simulink model "simu"  (R2014a)
settings: Solver=ode23t  StartTime=0.0  StopTime=2  FixedStep=0.00001  MaxStep=0.0001  RelTol=1e-3
undefined symbols (not defined in the file or in its folder): param
settings Model: Creator=Etienne  LastModifiedBy=Etienne

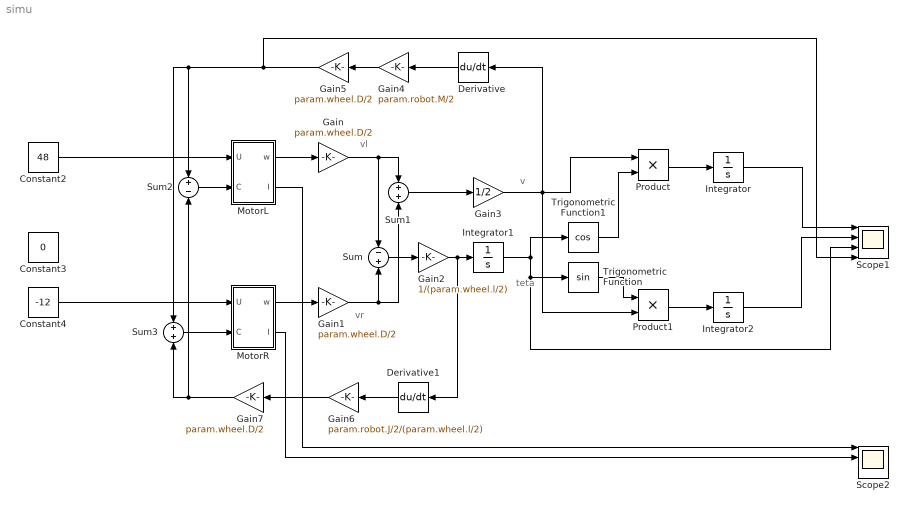
== system simu ==
  note: v
  note: teta
  note: vr
  note: vl
  Constant2 : Constant  Value=48
  Constant3 : Constant  Value=0
  Constant4 : Constant  Value=-12
  Derivative : Derivative
  Derivative1 : Derivative
  Gain{,1,5,7} (4 alike) : Gain  Gain=param.wheel.D/2
  Gain2 : Gain  Gain=1/(param.wheel.l/2)
  Gain3 : Gain  Gain=1/2
  Gain4 : Gain  Gain=param.robot.M/2
  Gain6 : Gain  Gain=param.robot.J/2/(param.wheel.l/2)
  Integrator : Integrator
  Integrator1 : Integrator
  Integrator2 : Integrator
  MotorL : Subsystem
  MotorR : Subsystem
  Product : Product
  Product1 : Product
  Scope1 : Scope  NumInputPorts=4
      settings: TimeRange=2  YMin=-0.06~-0.1~-15~-0.2  YMax=0.06~0.01999999999999999~0~1  MaxDataPoints=5000000
  Scope2 : Scope  NumInputPorts=4
      settings: TimeRange=2  YMin=0~-6~-1~-1  YMax=6~0~1~1  SaveName=ScopeData2  MaxDataPoints=5000000
  Sum : Sum  Inputs=-|+
  Sum1 : Sum  Inputs=+|+
  Sum2 : Sum  Inputs=+|-
  Sum3 : Sum  Inputs=+|+
  Trigonometric Function : Trigonometry
  Trigonometric Function1 : Trigonometry  Operator=cos
  wires:
  Gain/1 -> Sum/1, Sum1/1
  Integrator/1 -> Scope1/1
  MotorR/1(w) -> Gain1/1
  Gain1/1 -> Sum/2, Sum1/2
  Sum/1 -> Gain2/1
  Gain2/1 -> Derivative1/1, Integrator1/1
  Sum1/1 -> Gain3/1
  Gain3/1 -> Derivative/1, Product1/2, Product/1
  Integrator1/1 -> Trigonometric Function1/1, Scope1/3, Trigonometric Function/1
  Trigonometric Function1/1 -> Product/2
  Trigonometric Function/1 -> Product1/1
  Product/1 -> Integrator/1
  Product1/1 -> Integrator2/1
  Integrator2/1 -> Scope1/2
  Constant4/1 -> MotorR/1(U)
  Derivative/1 -> Gain4/1
  Gain4/1 -> Gain5/1
  Gain5/1 -> Sum3/1, Sum2/1, Scope1/4
  MotorR/2(I) -> Scope2/2
  Sum3/1 -> MotorR/2(C)
  Gain6/1 -> Gain7/1
  Gain7/1 -> Sum2/2, Sum3/2
  Derivative1/1 -> Gain6/1
  Constant2/1 -> MotorL/1(U)
  Sum2/1 -> MotorL/2(C)
  MotorL/1(w) -> Gain/1
  MotorL/2(I) -> Scope2/1

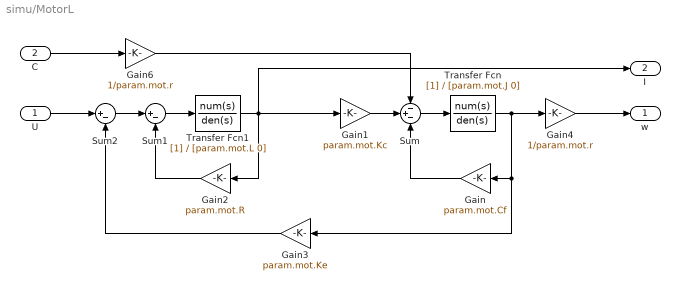
== system simu/MotorL ==
  U : Inport
  C : Inport  Port=2
  Gain : Gain  Gain=param.mot.Cf
  Gain1 : Gain  Gain=param.mot.Kc
  Gain2 : Gain  Gain=param.mot.R
  Gain3 : Gain  Gain=param.mot.Ke
  Gain4 : Gain  Gain=1/param.mot.r
  Gain6 : Gain  Gain=1/param.mot.r
  Sum : Sum  Inputs=-+-
  Sum1 : Sum  Inputs=|+-
  Sum2 : Sum  Inputs=|+-
  Transfer Fcn : TransferFcn  Denominator=[param.mot.J 0]
  Transfer Fcn1 : TransferFcn  Denominator=[param.mot.L 0]
  w : Outport
  I : Outport  Port=2
  wires:
  Gain1/1 -> Sum/2
  Transfer Fcn/1 -> Gain4/1, Gain3/1, Gain/1
  Gain3/1 -> Sum2/2
  Gain/1 -> Sum/3
  Sum2/1 -> Sum1/1
  Gain2/1 -> Sum1/2
  Sum1/1 -> Transfer Fcn1/1
  U/1 -> Sum2/1
  C/1 -> Gain6/1
  Gain6/1 -> Sum/1
  Gain4/1 -> w/1
  Sum/1 -> Transfer Fcn/1
  Transfer Fcn1/1 -> Gain1/1, I/1, Gain2/1

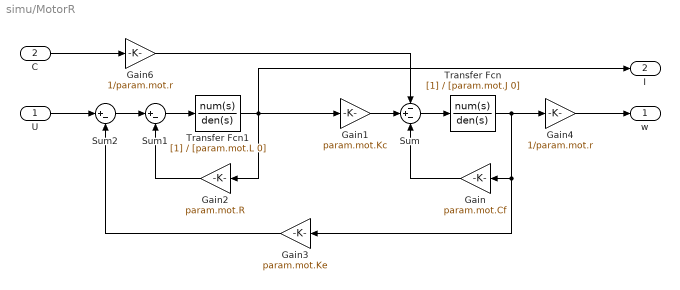
== system simu/MotorR ==
  U : Inport
  C : Inport  Port=2
  Gain : Gain  Gain=param.mot.Cf
  Gain1 : Gain  Gain=param.mot.Kc
  Gain2 : Gain  Gain=param.mot.R
  Gain3 : Gain  Gain=param.mot.Ke
  Gain4 : Gain  Gain=1/param.mot.r
  Gain6 : Gain  Gain=1/param.mot.r
  Sum : Sum  Inputs=-+-
  Sum1 : Sum  Inputs=|+-
  Sum2 : Sum  Inputs=|+-
  Transfer Fcn : TransferFcn  Denominator=[param.mot.J 0]
  Transfer Fcn1 : TransferFcn  Denominator=[param.mot.L 0]
  w : Outport
  I : Outport  Port=2
  wires:
  Gain1/1 -> Sum/2
  Transfer Fcn/1 -> Gain4/1, Gain3/1, Gain/1
  Gain3/1 -> Sum2/2
  Gain/1 -> Sum/3
  Sum2/1 -> Sum1/1
  Gain2/1 -> Sum1/2
  Sum1/1 -> Transfer Fcn1/1
  U/1 -> Sum2/1
  C/1 -> Gain6/1
  Gain6/1 -> Sum/1
  Gain4/1 -> w/1
  Sum/1 -> Transfer Fcn/1
  Transfer Fcn1/1 -> Gain1/1, I/1, Gain2/1
